simulink model "GalvoModel_v3_blockumbau_noCC"  (R2013a)
settings: Solver=ode45  StartTime=0.0  StopTime=20e-3  MaxStep=1e-6  RelTol=1e-3
values from neighbouring files (symbols this model uses):
  BEM = 108e-6    (= 0.000108)    [GalvoModel_thesis2_proc.m]
  CL = 180e-6    (= 0.00018)    [GalvoModel_thesis2_proc.m]    (also in GalvoModel_v4_sys.m = @(x,n) repmat(x, 1, n))
  CR = 2.79    [GalvoModel_thesis2_proc.m]
  FR = 4e-6    (= 4e-06)    [GalvoModel_thesis2_proc.m]
  KTR = 47e-3    (= 0.047)    [GalvoModel_thesis2_proc.m]
  RIN = 1.25e-8    (= 1.25e-08)    [GalvoModel_thesis2_proc.m]
  TRC = 6.17e-3    (= 0.00617)    [GalvoModel_thesis2_proc.m]
libraries: simulink x1
settings Model: Creator=mainster  LastModifiedBy=mainster
settings DebuggingCC: SolverPrmCheckMsg=none

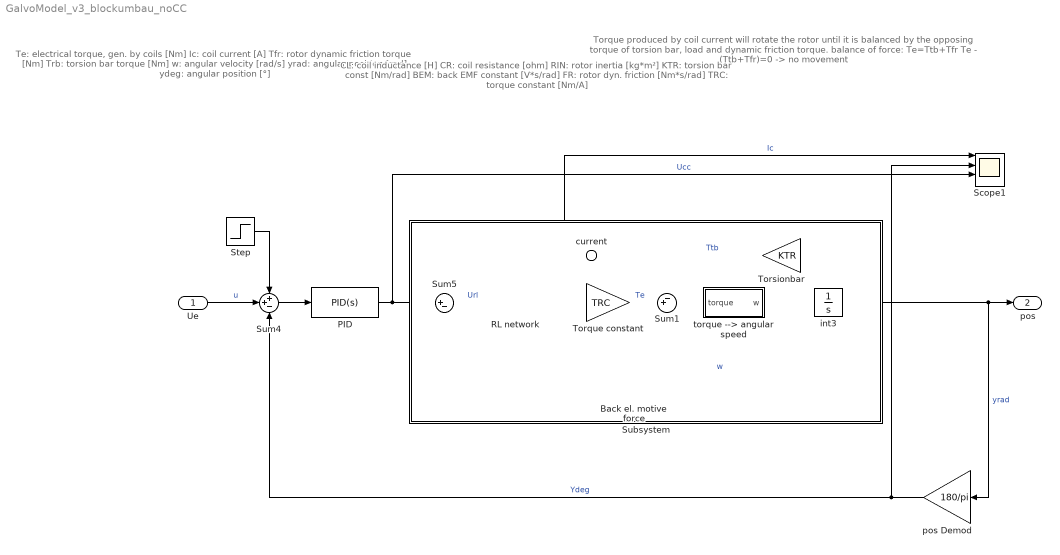
== system GalvoModel_v3_blockumbau_noCC ==
  note: Te: 	electrical torque, gen. by coils	[Nm]
      |  Ic: 	coil current							[A]
      |  Tfr:	rotor dynamic friction torque 		[Nm]
      |  Trb:	torsion bar torque					[Nm]
      |  w:		angular velocity 					[rad/s]
      |  yrad:	angular position 					[rad]
      |  ydeg:	angular position 					[°]
  note: Torque produced by coil current will rotate the rotor until
      | it is balanced by the opposing torque of torsion bar, load
      | and dynamic friction torque.
      | balance of force: 	Te=Ttb+Tfr
      | 						Te - (Ttb+Tfr)=0  ->  no movement
  note: CL:	coil inductance 		[H]
      |  CR:	coil resistance 		[ohm]
      |  RIN:	rotor inertia 			[kg*m²]
      |  KTR:	torsion bar const 	[Nm/rad]
      |  BEM:	back EMF constant	[V*s/rad]
      |  FR:	rotor dyn. friction	[Nm*s/rad]
      |  TRC:	torque constant		[Nm/A]
  Ue : Inport
  Back el. motive force : Gain  Gain=BEM
  PID : simulink/Continuous/PID Controller  Controller=PID  TimeDomain=Continuous-time  SampleTime=1  IntegratorMethod=Forward Euler  FilterMethod=Forward Euler  Form=Parallel  P=-2.27565518672585  I=-742.384468387289  D=-0.00145305427362546  N=1320192.31924849  InitialConditionSource=internal  InitialConditionForIntegrator=0  InitialConditionForFilter=0  ExternalReset=none  LimitOutput=on  UpperSaturationLimit=30  LowerSaturationLimit=-30  LinearizeAsGain=off  AntiWindupMode=none  Kb=1  TrackingMode=off  Kt=0  PParamMin=[]  PParamMax=[]  IParamMin=[]  IParamMax=[]  DParamMin=[]  DParamMax=[]  NParamMin=[]  NParamMax=[]  KbParamMin=[]  KbParamMax=[]  KtParamMin=[]  KtParamMax=[]  POutMin=[]  POutMax=[]  IOutMin=[]  IOutMax=[]  DOutMin=[]  DOutMax=[]  NOutMin=[]  NOutMax=[]  KbOutMin=[]  KbOutMax=[]  KtOutMin=[]  KtOutMax=[]  IntegratorOutMin=[]  IntegratorOutMax=[]  FilterOutMin=[]  FilterOutMax=[]  SumOutMin=[]  SumOutMax=[]  SumI1OutMin=[]  SumI1OutMax=[]  SumI2OutMin=[]  SumI2OutMax=[]  SumI3OutMin=[]  SumI3OutMax=[]  SumDOutMin=[]  SumDOutMax=[]  SaturationOutMin=[]  SaturationOutMax=[]  IntegratorContinuousStateAttributes=''  IntegratorStateMustResolveToSignalObject=off  IntegratorRTWStateStorageClass=Auto  FilterContinuousStateAttributes=''  FilterStateMustResolveToSignalObject=off  FilterRTWStateStorageClass=Auto
  RL network : Subsystem
  Scope1 : Scope  NumInputPorts=4
      settings: ShowLegends=on  TimeRange=0.02  YMin=-0.4~0~-10~-1  YMax=0.6~4~2~1  MaxDataPoints=500000
  Step : Step  Time=1e-3  After=15  SampleTime=0
      settings: AttributesFormatString=Ampl.: %<After>
  Subsystem : Subsystem  mask{d=0}
      mask Display: disp('')
  Sum1 : Sum  Inputs=-+|
  Sum4 : Sum  Inputs=++-
  Sum5 : Sum  Inputs=|+-
  Torque constant : Gain  Gain=TRC
  Torsionbar : Gain  Gain=KTR
  int3 : Integrator
  pos Demod : Gain  Gain=180/pi
  torque --> angular speed : Subsystem
  current : Outport
  pos : Outport  Port=2
  wires:
  int3/1 -> pos Demod/1, pos/1, Torsionbar/1  "yrad"
  Torque constant/1 -> Sum1/2  "Te"
  Back el. motive force/1 -> Sum5/2
  Sum4/1 -> PID/1
  Sum5/1 -> RL network/1(Ucl)  "Url"
  RL network/1(Ic) -> Scope1/1, current/1, Torque constant/1  "Ic"
  Torsionbar/1 -> Sum1/1  "Ttb"
  torque --> angular speed/1(w) -> Back el. motive force/1, int3/1  "w"
  Sum1/1 -> torque --> angular speed/1(torque)
  Step/1 -> Sum4/1
  Ue/1 -> Sum4/2  "u"
  pos Demod/1 -> Sum4/3, Scope1/2  "Ydeg"
  PID/1 -> Sum5/1, Scope1/3  "Ucc"

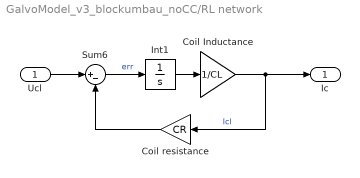
== system GalvoModel_v3_blockumbau_noCC/RL network ==
  Ucl : Inport
  Coil Inductance : Gain  Gain=1/CL
  Coil resistance : Gain  Gain=CR
  Int1 : Integrator
  Sum6 : Sum  Inputs=|+-
      settings: AttributesFormatString=%<Name>
  Ic : Outport
  wires:
  Int1/1 -> Coil Inductance/1
  Coil resistance/1 -> Sum6/2
  Coil Inductance/1 -> Ic/1, Coil resistance/1  "Icl"
  Ucl/1 -> Sum6/1
  Sum6/1 -> Int1/1  "err"

== system GalvoModel_v3_blockumbau_noCC/Subsystem ==

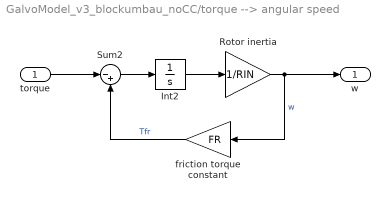
== system GalvoModel_v3_blockumbau_noCC/torque --> angular speed ==
  torque : Inport
  Int2 : Integrator
  Rotor inertia : Gain  Gain=1/RIN
  Sum2 : Sum  Inputs=|-+
  friction torque constant : Gain  Gain=FR
  w : Outport
  wires:
  Int2/1 -> Rotor inertia/1
  Sum2/1 -> Int2/1
  Rotor inertia/1 -> w/1, friction torque constant/1  "w"
  torque/1 -> Sum2/1
  friction torque constant/1 -> Sum2/2  "Tfr"
